simulink model "mat"  (R2019a)
settings: Solver=VariableStepAuto  StartTime=0.0  StopTime=10  RelTol=1e-3
settings Model: Creator=MOSTFA KHALID  LastModifiedBy=moham

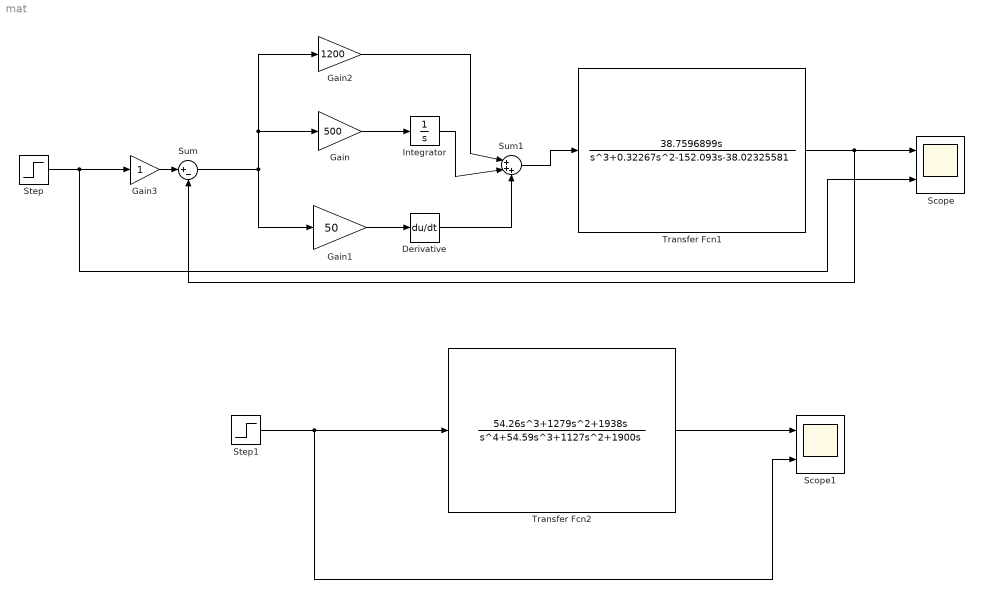
== system mat ==
  Derivative : Derivative
  Gain : Gain  Gain=500
  Gain1 : Gain  Gain=50
  Gain2 : Gain  Gain=1200
  Gain3 : Gain
  Integrator : Integrator
  Scope : Scope  NumInputPorts=2
  Scope1 : Scope  NumInputPorts=2
  Step : Step  SampleTime=0
  Step1 : Step  SampleTime=0
  Sum : Sum  Inputs=|+-
  Sum1 : Sum  Inputs=|+++
  Transfer Fcn1 : TransferFcn  Numerator=[38.7596899 0]  Denominator=[1 0.32267 -152.093 -38.02325581 ]
  Transfer Fcn2 : TransferFcn  Numerator=[54.26 1279 1938 0]  Denominator=[1 54.59 1127 1900 0 ]
  wires:
  Gain/1 -> Integrator/1
  Gain1/1 -> Derivative/1
  Gain2/1 -> Sum1/1
  Integrator/1 -> Sum1/2
  Derivative/1 -> Sum1/3
  Gain3/1 -> Sum/1
  Transfer Fcn1/1 -> Scope/1, Sum/2
  Step/1 -> Scope/2, Gain3/1
  Sum/1 -> Gain2/1, Gain/1, Gain1/1
  Sum1/1 -> Transfer Fcn1/1
  Step1/1 -> Transfer Fcn2/1, Scope1/2
  Transfer Fcn2/1 -> Scope1/1
